simulink model "DIavecTOT"  (R2017a)
settings: Solver=VariableStepAuto  StartTime=0.0  StopTime=30  RelTol=1e-3
settings Model: Creator=pc  LastModifiedBy=pc

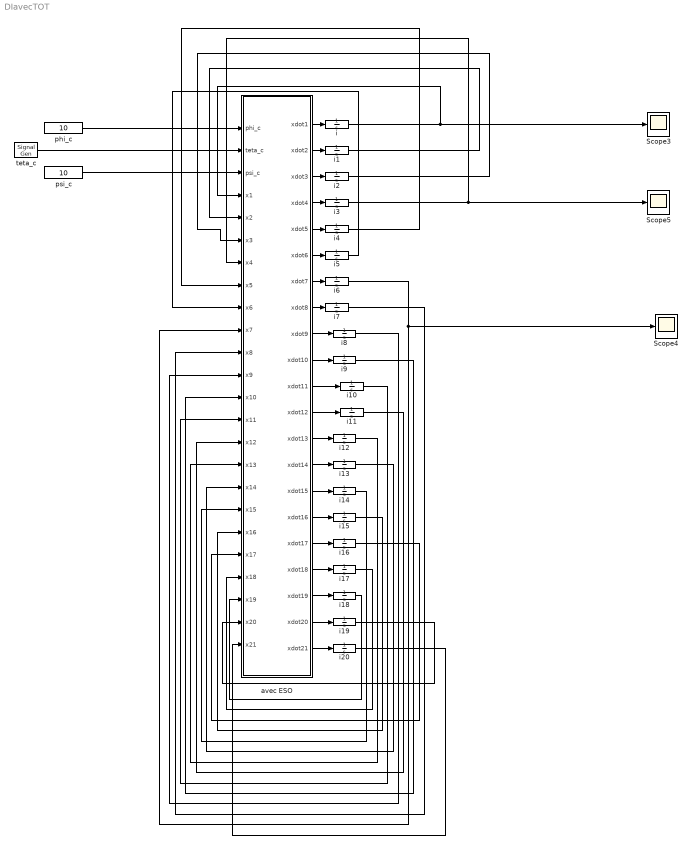
== system DIavecTOT ==
  Scope3 : Scope
  Scope4 : Scope
  Scope5 : Scope
  avec ESO : MATLAB Function  TreatAsAtomicUnit=on
  i{,1..20} (21 alike) : Integrator
  phi_c : Constant  Value=10
  psi_c : Constant  Value=10
  teta_c : SignalGenerator  WaveForm=square  Amplitude=10  Frequency=0.1
  wires:
  phi_c/1 -> avec ESO/1(phi_c)
  teta_c/1 -> avec ESO/2(teta_c)
  psi_c/1 -> avec ESO/3(psi_c)
  avec ESO/1(xdot1) -> i/1
  i/1 -> avec ESO/4(x1), Scope3/1
  avec ESO/2(xdot2) -> i1/1
  avec ESO/3(xdot3) -> i2/1
  avec ESO/4(xdot4) -> i3/1
  avec ESO/5(xdot5) -> i4/1
  avec ESO/6(xdot6) -> i5/1
  avec ESO/7(xdot7) -> i6/1
  avec ESO/8(xdot8) -> i7/1
  avec ESO/9(xdot9) -> i8/1
  avec ESO/10(xdot10) -> i9/1
  avec ESO/11(xdot11) -> i10/1
  avec ESO/12(xdot12) -> i11/1
  avec ESO/13(xdot13) -> i12/1
  avec ESO/14(xdot14) -> i13/1
  avec ESO/15(xdot15) -> i14/1
  avec ESO/16(xdot16) -> i15/1
  avec ESO/17(xdot17) -> i16/1
  avec ESO/18(xdot18) -> i17/1
  avec ESO/19(xdot19) -> i18/1
  avec ESO/20(xdot20) -> i19/1
  avec ESO/21(xdot21) -> i20/1
  i20/1 -> avec ESO/24(x21)
  i19/1 -> avec ESO/23(x20)
  i18/1 -> avec ESO/22(x19)
  i17/1 -> avec ESO/21(x18)
  i16/1 -> avec ESO/20(x17)
  i15/1 -> avec ESO/19(x16)
  i14/1 -> avec ESO/18(x15)
  i13/1 -> avec ESO/17(x14)
  i12/1 -> avec ESO/16(x13)
  i11/1 -> avec ESO/15(x12)
  i10/1 -> avec ESO/14(x11)
  i9/1 -> avec ESO/13(x10)
  i8/1 -> avec ESO/12(x9)
  i7/1 -> avec ESO/11(x8)
  i6/1 -> Scope4/1, avec ESO/10(x7)
  i5/1 -> avec ESO/9(x6)
  i4/1 -> avec ESO/8(x5)
  i3/1 -> avec ESO/7(x4), Scope5/1
  i2/1 -> avec ESO/6(x3)
  i1/1 -> avec ESO/5(x2)

== matlab function DIavecTOT/avec ESO ==
  data: phi_c input; teta_c input; psi_c input; xdot1 output; x1 input; x2 input; x3 input; x4 input; x5 input; x6 input; x7 input; x8 input; x9 input; x10 input; x11 input; x12 input; x13 input; x14 input; x15 input; x16 input; x17 input; x18 input; x19 input; x20 input; x21 input; xdot2 output; xdot3 output; xdot4 output; xdot5 output; xdot6 output; xdot7 output; xdot8 output; xdot9 output; xdot10 output; xdot11 output; xdot12 output; xdot13 output; xdot14 output; xdot15 output; xdot16 output; xdot17 output; xdot18 output; xdot19 output; xdot20 output; xdot21 output
function [xdot1,xdot2,xdot3,xdot4,xdot5,xdot6,xdot7,xdot8,xdot9,xdot10,xdot11,xdot12,xdot13,xdot14,xdot15,xdot16,xdot17,xdot18,xdot19,xdot20,xdot21] = fcn(phi_c,teta_c,psi_c,x1,x2,x3,x4,x5,x6,x7,x8,x9,x10,x11,x12,x13,x14,x15,x16,x17,x18,x19,x20,x21)
alfa1=0.9; alfa2=0.3;
delta=0.1;
kd1=6.4;kd2=6.4;kd3=6.4;
kp1=16;kp2=16;kp3=16;
beta1=100; beta2=3000; beta3=5000;
%--------------------------------------------------------------------------
Ix=22682;
Iy=77095;
Iz=95561;
Ixz=1125;
SOM=Ix*Iz-Ixz^2;
c1=((Iy-Iz)*Iz-Ixz^2)/SOM;
c2=((Ix-Iy+Iz)*Ixz)/SOM;
c3=Iz/SOM;
c4=Ixz/SOM;
c5=(Iz-Ix)/Iy;
c6=Ixz/Iy;
c7=1/Iy;
c8=(Ix*(Ix-Iy)+Ixz^2)/SOM;
c9=Ix/SOM;
%--------------------------------------------------------------------------
phi=x1;
teta=x4;
p=x19;
r=x20;
q=x21;
%--------------------------------------------------------------------------
B=[c3+c4*cosd(phi)*tand(teta),c7*sind(phi)*tand(teta),c4+c9*cosd(phi)*tand(teta);
    -c4*sind(phi),c7*cosd(phi),-c9*sind(phi);
    c4*cosd(phi)*(1/cosd(teta)),c7*sind(phi)*(1/cosd(teta)),c9*cosd(phi)*(1/cosd(teta))];
phidot=p+tand(teta)*(q*sind(phi)+r*cosd(phi));
tetadot=q*cosd(phi)-r*sind(phi);
A1=((c1*r+c2*p)*q)+(tetadot/cosd(teta)^2)*(q*sind(phi)+r*cosd(phi))+tand(teta)*((c5*p*r-c6*(p^2-r^2))*sind(phi)+q*(phidot*cosd(phi))+((c8*p-c2*r)*q)*cosd(phi)-r*phidot*sind(phi));
A2=(c5*p*r-c6*(p^2-r^2))*cosd(phi)-phidot*sind(phi)*q-(((c8*p-c2*r)*q)*sind(phi)+phidot*cosd(phi)*r);
A3=((c5*p*r-c6*(p^2-r^2))*sind(phi)+phidot*cosd(phi)*q+((c8*p-c2*r)*q)*cosd(phi)-phidot*sind(phi)*r)*cosd(teta)/cosd(teta)^2+(tetadot*sind(teta)*(q*sind(phi)+r*cosd(phi)))/cosd(teta)^2;
%--------------------------------------------------------------------------
pp=inv(B);
L=pp(1,:)*[(kp1*phi_c-x12)-A1;(kp2*teta_c-x15)-A2;(kp3*psi_c-x18)-A3];
M=pp(2,:)*[(kp1*phi_c-x12)-A1;(kp2*teta_c-x15)-A2;(kp3*psi_c-x18)-A3];
N=pp(3,:)*[(kp1*phi_c-x12)-A1;(kp2*teta_c-x15)-A2;(kp3*psi_c-x18)-A3];
%************------************----------**************-----------------
e=x10-x1;                                     %y(1)=phi y(10)=Z1_phi 
e2=x13-x4;                                      %y(4)=teta y(14)=Z1_teta
e3=x16-x7;                                      %y(7)=psi y(16)=Z1_PSI
%************------************----------**************-----------------
xdot1=x2;   
%xdot2=A1+B(1,:)*[L;M;N];
xdot2=x3+kp1*phi_c;
%xdot3=A1dot+Bdot(1,:)*u+B(1,:)*udot;
Delta_u1=x12+kp1*x1+kd1*x2;
xdot3=-kp1*x2-kd1*(x3+kp1*phi_c)-Delta_u1;
%---ESO1 Z_PHI---
xdot10=x11-beta1*e;                           %y(11)=Z2_phi
%^^^^^^^^^^^^^^^^^^^^^^^^^^^^^^^^^^^^^^^^^^^^^^^^^^^^^^^^^^^^^^^^^^^^^^^^^^
if abs(e)> delta 
FAL=abs(e)^alfa1*sign(e);
xdot11=x12-beta2*FAL+kp1*phi_c;%y(12)=Z3_phi
else 
    FAL=e/(delta^(1-alfa1));
 xdot11=x12-beta2*FAL+kp1*phi_c;%y(12)=Z3_phi
end
%^^^^^^^^^^^^^^^^^^^^^^^^^^^^^^^^^^^^^^^^^^^^^^^^^^^^^^^^^^^^^^^^^^^^^^^^^^ 
if abs(e)> delta 
FAL1=abs(e)^alfa2*sign(e);
xdot12=-beta3*FAL1;
else 
    FAL1=e/(delta^(1-alfa2));
    xdot12=-beta3*FAL1;
end
%^^^^^^^^^^^^^^^^^^^^^^^^^^^^^^^^^^^^^^^^^^^^^^^^^^^^^^^^^^^^^^^^^^^^^^^^^^


%--------------------------------------------------------------------------
xdot4=x5;   
%xdot4=A2+B(2,:)*[L;M;N];  
xdot5=x6+kp2*teta_c;
%xdot6=A2dot+Bdot(2,:)*u+B(2,:)*udot;
Delta_u2=x15+kp2*x4+kd2*x5;
xdot6=-kp2*x5-kd1*(x6+kp2*teta_c)-Delta_u2;
%---ESO2 Z_Teta---
xdot13=x14-beta1*e2;                            %y(15)=Z2_teta
%^^^^^^^^^^^^^^^^^^^^^^^^^^^^^^^^^^^^^^^^^^^^^^^^^^^^^^^^^^^^^^^^^^^^^^^^^^
if abs(e2)> delta 
FAL2=abs(e2)^alfa1*sign(e2);
xdot14=x15-beta2*FAL2+kp2*teta_c;%y(16)=Z3_teta 
else
    FAL2=e2/(delta^(1-alfa1));
xdot14=x15-beta2*FAL2+kp2*teta_c;%y(16)=Z3_teta 
end
%^^^^^^^^^^^^^^^^^^^^^^^^^^^^^^^^^^^^^^^^^^^^^^^^^^^^^^^^^^^^^^^^^^^^^^^^^^ 
if abs(e2)> delta 
FAL3=abs(e2)^alfa2*sign(e2);
xdot15=-beta3*FAL3;
else
    FAL3=e2/(delta^(1-alfa2));
xdot15=-beta3*FAL3;
end
%^^^^^^^^^^^^^^^^^^^^^^^^^^^^^^^^^^^^^^^^^^^^^^^^^^^^^^^^^^^^^^^^^^^^^^^^^^


%--------------------------------------------------------------------------
xdot7=x8;   
%xdot6=A3+B(3,:)*[L;M;N];
xdot8=x9+kp3*psi_c;
%xdot9=A3dot+Bdot(3,:)*u+B(3,:)*udot;
Delta_u3=x18+kp3*x7+kd3*x8;
xdot9=-kp3*x8-kd3*(x9+kp3*psi_c)-Delta_u3;
%---ESO3 Z_PSI---
xdot16=x17-beta1*e3;                          %y(17)=Z2_PSI
%^^^^^^^^^^^^^^^^^^^^^^^^^^^^^^^^^^^^^^^^^^^^^^^^^^^^^^^^^^^^^^^^^^^^^^^^^^
if abs(e3)> delta 
FAL4=abs(e3)^alfa1*sign(e3);
xdot17=x18-beta2*FAL4+kp3*psi_c; %y(18)=Z3_PSI
else
    FAL4=e3/(delta^(1-alfa1));
xdot17=x18-beta2*FAL4+kp3*psi_c; %y(18)=Z3_PSI
end
%^^^^^^^^^^^^^^^^^^^^^^^^^^^^^^^^^^^^^^^^^^^^^^^^^^^^^^^^^^^^^^^^^^^^^^^^^^ 
if abs(e3)> delta 
FAL5=abs(e3)^alfa2*sign(e3);
xdot18=-beta3*FAL5;
else
    FAL5=e3/(delta^(1-alfa2));
xdot18=-beta3*FAL5;
end
%^^^^^^^^^^^^^^^^^^^^^^^^^^^^^^^^^^^^^^^^^^^^^^^^^^^^^^^^^^^^^^^^^^^^^^^^^^

%--------------------------------------------------------------------------
xdot19=(c1*r+c2*p)*q+c3*L+c4*N;  %=pdot
xdot20=(c8*p-c2*r)*q+c4*L+c9*N;  %=rdot
xdot21=c5*p*r-c6*(p^2-r^2)+c7*M; %=qdot
end
